simulink model "hardware_deployment"  (R2021a)
settings: Solver=VariableStepAuto  StartTime=0.0  StopTime=10.0  RelTol=1e-3
undefined symbols (not defined in the file or in its folder): ADCResolution, ADCSamplingFrequency, AnalogReference
libraries: c2802xlib x4
settings Model: Creator=61301765  LastModifiedBy=61301765

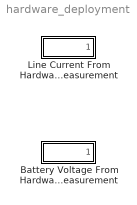
== system hardware_deployment ==
  Battery Voltage From Hardware Measurement : Subsystem
  Line Current From Hardware Measurement : Subsystem

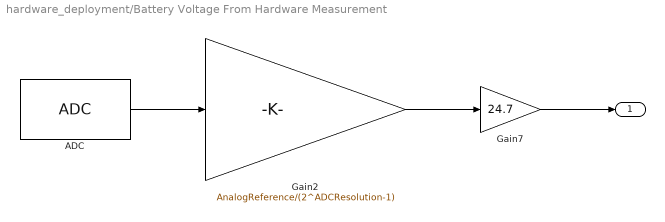
== system hardware_deployment/Battery Voltage From Hardware Measurement ==
  ADC : c2802xlib/ADC  blkParamProc=C2000_Type5  ADCModule=A  samplingMode=Single sample mode  ADCResolution=12-bit (Single-ended input)  useSOC1=SOC3  useSOC2=SOC0_SOC1  SOCAcquisitionWindow=8  SOCTriggerSource=Software  SOCInterruptTrigger=No ADCINT  Ts=1/ADCSamplingFrequency  dType=double  postInterrupt=off  interruptSel=ADCINT1  ADCINTContinuous=on  endma=off  chdma=1  conv1=ADCINA0  conv2=ADCINA0 and ADCINB0  conv1_Type4=ADCIN0  conv2_Type4=ADCIN0 and ADCIN1
  Gain2 : Gain  Gain=AnalogReference/(2^ADCResolution-1)
  Gain7 : Gain  Gain=24.7
  " " : Outport
  wires:
  Gain7/1 -> " "/1
  Gain2/1 -> Gain7/1
  ADC/1 -> Gain2/1

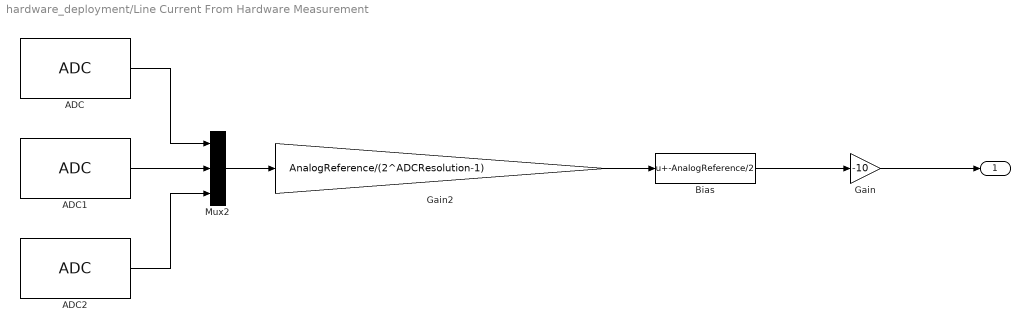
== system hardware_deployment/Line Current From Hardware Measurement ==
  ADC : c2802xlib/ADC  blkParamProc=C2000_Type5  ADCModule=A  samplingMode=Single sample mode  ADCResolution=12-bit (Single-ended input)  useSOC1=SOC0  useSOC2=SOC0_SOC1  SOCAcquisitionWindow=8  SOCTriggerSource=Software  SOCInterruptTrigger=No ADCINT  Ts=1/ADCSamplingFrequency  dType=double  postInterrupt=off  interruptSel=ADCINT1  ADCINTContinuous=on  endma=off  chdma=1  conv1=ADCINA0  conv2=ADCINA0 and ADCINB0  conv1_Type4=ADCIN0  conv2_Type4=ADCIN0 and ADCIN1
  ADC1 : c2802xlib/ADC  blkParamProc=C2000_Type5  ADCModule=A  samplingMode=Single sample mode  ADCResolution=12-bit (Single-ended input)  useSOC1=SOC1  useSOC2=SOC0_SOC1  SOCAcquisitionWindow=8  SOCTriggerSource=Software  SOCInterruptTrigger=No ADCINT  Ts=1/ADCSamplingFrequency  dType=double  postInterrupt=off  interruptSel=ADCINT1  ADCINTContinuous=on  endma=off  chdma=1  conv1=ADCINA0  conv2=ADCINA0 and ADCINB0  conv1_Type4=ADCIN0  conv2_Type4=ADCIN0 and ADCIN1
  ADC2 : c2802xlib/ADC  blkParamProc=C2000_Type5  ADCModule=A  samplingMode=Single sample mode  ADCResolution=12-bit (Single-ended input)  useSOC1=SOC2  useSOC2=SOC0_SOC1  SOCAcquisitionWindow=8  SOCTriggerSource=Software  SOCInterruptTrigger=No ADCINT  Ts=1/ADCSamplingFrequency  dType=double  postInterrupt=off  interruptSel=ADCINT1  ADCINTContinuous=on  endma=off  chdma=1  conv1=ADCINA0  conv2=ADCINA0 and ADCINB0  conv1_Type4=ADCIN0  conv2_Type4=ADCIN0 and ADCIN1
  Bias : Bias  Bias=-AnalogReference/2
  Gain : Gain  Gain=-10
  Gain2 : Gain  Gain=AnalogReference/(2^ADCResolution-1)
  Mux2 : Mux  Inputs=3
  " " : Outport
  wires:
  Gain2/1 -> Bias/1
  ADC/1 -> Mux2/1
  ADC2/1 -> Mux2/3
  ADC1/1 -> Mux2/2
  Mux2/1 -> Gain2/1
  Bias/1 -> Gain/1
  Gain/1 -> " "/1
